simulink model "Task_2"  (R2023b)
settings: Solver=ode4  StartTime=t0  StopTime=tf  FixedStep=dt  RelTol=1e-3
values from neighbouring files (symbols this model uses):
  F_vect = [8; 5; 4]    [Task1_RK4.m]    (also in get_states_dot.m)
  M_vect = [5; 10; 20]    [Task1_RK4.m]    (also in get_states_dot.m)
libraries: shared6dof x1, dspsigops x1
settings Model: Creator=Saif Mohamed  LastModifiedBy=Saif Mohamed

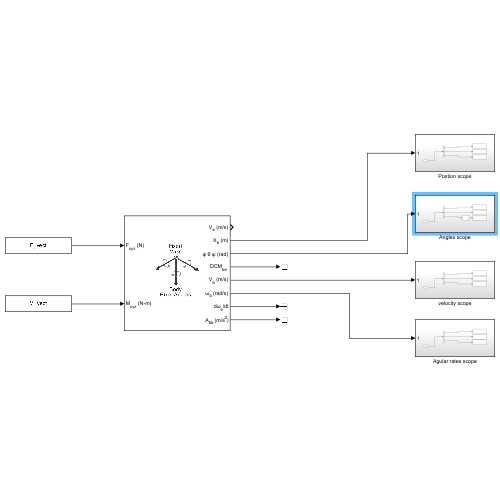
[thumbnail: Simulink's stored preview of the top-level diagram]
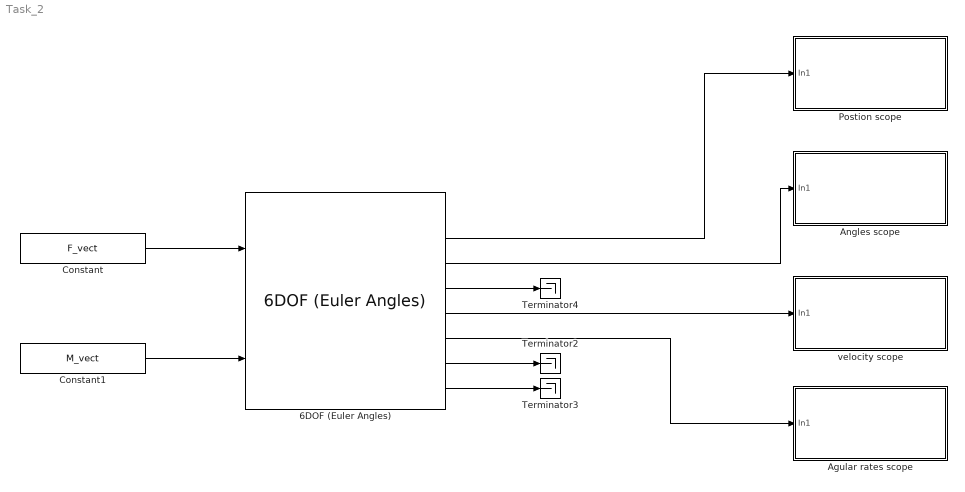
== system Task_2 ==
  6DOF (Euler Angles) : shared6dof/6DOF (Euler Angles)  units=Metric (MKS)  mtype=Fixed  rep=Euler Angles  xme_0=[2 4 7]  Vm_0=[10 2 0]  eul_0=[20*pi/180 15*pi/180 30*pi/180]  pm_0=[2*pi/180 1*pi/180 0]  mass_0=m  mass_e=0.5  mass_f=2.0  inertia=I_matrix  inertia_e=eye(3)  inertia_f=2*eye(3)  k_quat=1.0  vre_flag=on  abi_flag=off  aMode=0  xme_statename=''  Vm_statename=''  eul_statename=''  quat_statename=''  pm_statename=''  mass_statename=''
  Agular rates scope : Subsystem
  Angles scope : Subsystem
  Constant : Constant  Value=F_vect
  Constant1 : Constant  Value=M_vect
  Postion scope : Subsystem
  Terminator2 : Terminator
  Terminator3 : Terminator
  Terminator4 : Terminator
  velocity scope : Subsystem
  wires:
  Constant/1 -> 6DOF (Euler Angles)/1
  Constant1/1 -> 6DOF (Euler Angles)/2
  6DOF (Euler Angles)/2 -> Postion scope/1(In1)
  6DOF (Euler Angles)/3 -> Angles scope/1(In1)
  6DOF (Euler Angles)/6 -> Agular rates scope/1(In1)
  6DOF (Euler Angles)/7 -> Terminator2/1
  6DOF (Euler Angles)/8 -> Terminator3/1
  6DOF (Euler Angles)/4 -> Terminator4/1
  6DOF (Euler Angles)/5 -> velocity scope/1(In1)

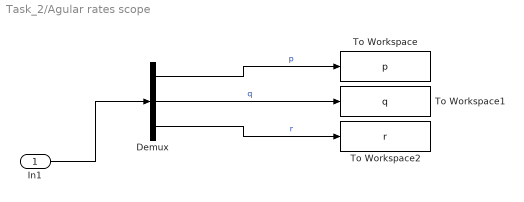
== system Task_2/Agular rates scope ==
  In1 : Inport
  Demux : Demux  Outputs=3
  To Workspace : ToWorkspace  VariableName=p  SampleTime=-1
  To Workspace1 : ToWorkspace  VariableName=q  SampleTime=-1
  To Workspace2 : ToWorkspace  VariableName=r  SampleTime=-1
  wires:
  In1/1 -> Demux/1
  Demux/2 -> To Workspace1/1  "q"
  Demux/1 -> To Workspace/1  "p"
  Demux/3 -> To Workspace2/1  "r"

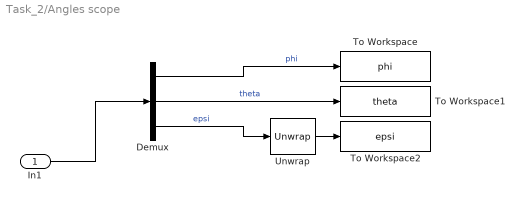
== system Task_2/Angles scope ==
  In1 : Inport
  Demux : Demux  Outputs=3
  To Workspace : ToWorkspace  VariableName=phi  SampleTime=-1
  To Workspace1 : ToWorkspace  VariableName=theta  SampleTime=-1
  To Workspace2 : ToWorkspace  VariableName=epsi  SampleTime=-1
  Unwrap : dspsigops/Unwrap  tol=pi  running=off
  wires:
  Demux/3 -> Unwrap/1  "epsi"
  Demux/1 -> To Workspace/1  "phi"
  Demux/2 -> To Workspace1/1  "theta"
  In1/1 -> Demux/1
  Unwrap/1 -> To Workspace2/1

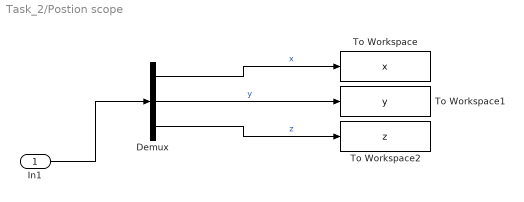
== system Task_2/Postion scope ==
  In1 : Inport
  Demux : Demux  Outputs=3
  To Workspace : ToWorkspace  VariableName=x  SampleTime=-1
  To Workspace1 : ToWorkspace  VariableName=y  SampleTime=-1
  To Workspace2 : ToWorkspace  VariableName=z  SampleTime=-1
  wires:
  In1/1 -> Demux/1
  Demux/2 -> To Workspace1/1  "y"
  Demux/1 -> To Workspace/1  "x"
  Demux/3 -> To Workspace2/1  "z"

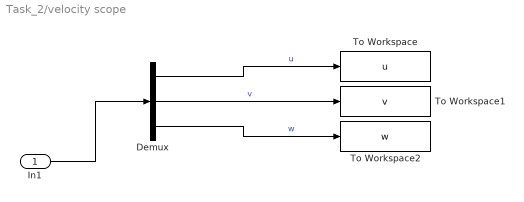
== system Task_2/velocity scope ==
  In1 : Inport
  Demux : Demux  Outputs=3
  To Workspace : ToWorkspace  VariableName=u  SampleTime=-1
  To Workspace1 : ToWorkspace  VariableName=v  SampleTime=-1
  To Workspace2 : ToWorkspace  VariableName=w  SampleTime=-1
  wires:
  Demux/3 -> To Workspace2/1  "w"
  Demux/1 -> To Workspace/1  "u"
  Demux/2 -> To Workspace1/1  "v"
  In1/1 -> Demux/1
